simulink model "NCarState"  (R2024b)
settings: Solver=FixedStepDiscrete  StartTime=0.0  StopTime=1  FixedStep=0.001  RelTol=1e-3  EnableMultiTasking=on
settings Model: DataDictionary=Master_Dictionary.sldd  EnableAccessToBaseWorkspace=off  Creator=torni  LastModifiedBy=oxbro
settings SolverCC: AlgebraicLoopSolver=TrustRegion
settings DataIOCC: ReturnWorkspaceOutputs=off
settings OptimizationCC: DefaultParameterBehavior=Inlined  EnhancedBackFolding=on  PassReuseOutputArgsAs=Individual arguments  ZeroExternalMemoryAtStartup=off  ZeroInternalMemoryAtStartup=off  MaxStackSize=512  OptimizeBlockOrder=speed  DifferentSizesBufferReuse=on  OptimizationCustomize=off  EfficientTunableParamExpr=on
settings DebuggingCC: ParameterTunabilityLossMsg=error  UnconnectedInputMsg=warning  UnconnectedOutputMsg=warning  UnconnectedLineMsg=warning  ArithmeticOperatorsInVariantConditions=warning
settings HardwareCC: ProdBitPerPointer=32  ProdBitPerSizeT=32  ProdBitPerPtrDiffT=32  ProdLargestAtomicInteger=Long  ProdLargestAtomicFloat=Double  ProdWordSize=32  ProdLongLongMode=on  ProdHWDeviceType=ARM Compatible->ARM Cortex-M
settings ModelReferenceCC: EnableRefExpFcnMdlSchedulingChecks=on
settings SFSimCC: MATLABDynamicMemAlloc=off  CustomCodeUndefinedFunction=UseInterfaceOnly
settings RTWCC: Description=Embedded Coder  SystemTargetFile=ert.tlc  HardwareBoard=STM32H7xx Based (Single-core)  TemplateMakefile=ert_default_tmf  CustomHeaderCode="#include \"stm32h7xx_ll_tim.h\""  CustomInitializer=LL_TIM_EnableCounter(TIM2);  Toolchain=GNU Tools for ARM Embedded Processors  GPUComputeCapability=3.5
settings CodeAppCC: ForceParamTrailComments=on  IgnoreCustomStorageClasses=off  OperatorAnnotations=on  SimulinkDataObjDesc=on  SFDataObjDesc=on  InsertBlockDesc=on
settings ERTTargetCC: TargetLangStandard=C99 (ISO)  CodeReplacementLibrary=ARM Cortex-M  ExtModeTransport=3  ExtModeStaticAlloc=on  ExtModeStaticAllocSize=2048  ExtModeMexFile=ext_xcp  ExtModeIntrfLevel=Level2 - Open

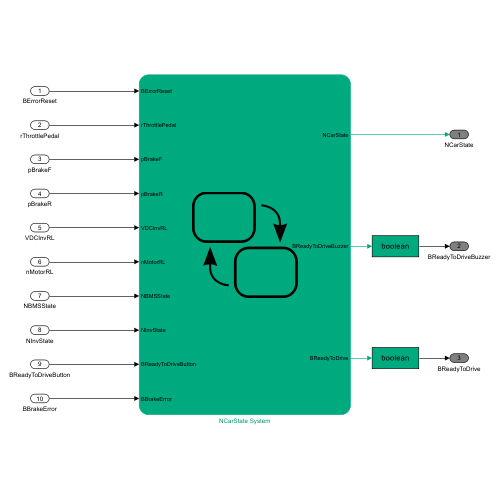
[thumbnail: Simulink's stored preview of the top-level diagram]
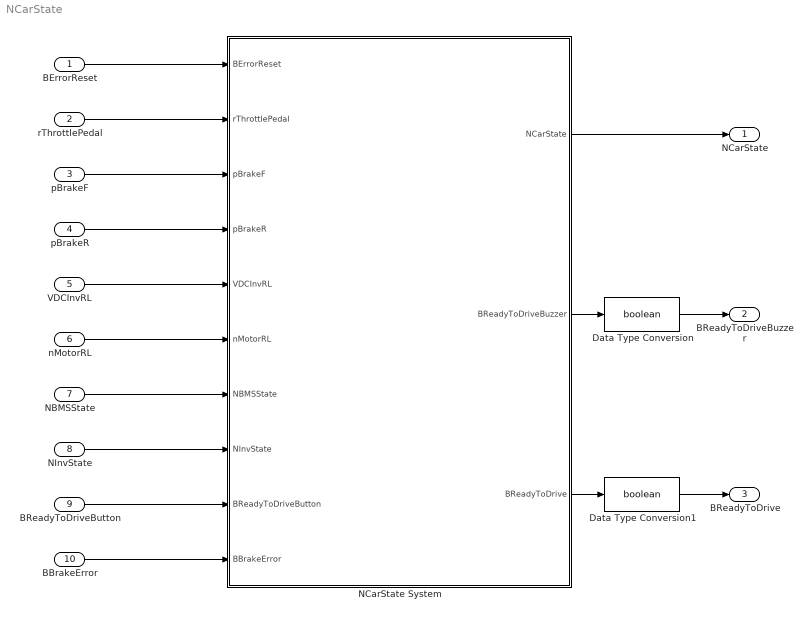
== system NCarState ==
  "BErrorReset " : Inport  OutDataTypeStr=boolean
  "rThrottlePedal " : Inport  Port=2  OutDataTypeStr=double
  "pBrakeF " : Inport  Port=3  OutDataTypeStr=double
  "pBrakeR " : Inport  Port=4  OutDataTypeStr=double
  VDCInvRL : Inport  Port=5  OutDataTypeStr=double
  "nMotorRL " : Inport  Port=6  OutDataTypeStr=double
  NBMSState : Inport  Port=7  OutDataTypeStr=double
  NInvState : Inport  Port=8  OutDataTypeStr=double
  BReadyToDriveButton : Inport  Port=9  OutDataTypeStr=boolean
  BBrakeError : Inport  Port=10  OutDataTypeStr=boolean
  Data Type Conversion : DataTypeConversion  OutDataTypeStr=boolean  SaturateOnIntegerOverflow=off  RndMeth=Floor
  Data Type Conversion1 : DataTypeConversion  OutDataTypeStr=boolean  SaturateOnIntegerOverflow=off  RndMeth=Floor
  NCarState System : Stateflow chart  TreatAsAtomicUnit=on
  NCarState : Outport  OutDataTypeStr=double  VectorParamsAs1DForOutWhenUnconnected=off
  BReadyToDriveBuzzer : Outport  Port=2  OutDataTypeStr=boolean  VectorParamsAs1DForOutWhenUnconnected=off
  BReadyToDrive : Outport  Port=3  OutDataTypeStr=boolean  VectorParamsAs1DForOutWhenUnconnected=off
  wires:
  "nMotorRL "/1 -> NCarState System/6(nMotorRL)
  "BErrorReset "/1 -> NCarState System/1(BErrorReset)
  "rThrottlePedal "/1 -> NCarState System/2(rThrottlePedal)
  "pBrakeR "/1 -> NCarState System/4(pBrakeR)
  VDCInvRL/1 -> NCarState System/5(VDCInvRL)
  "pBrakeF "/1 -> NCarState System/3(pBrakeF)
  NBMSState/1 -> NCarState System/7(NBMSState)
  NInvState/1 -> NCarState System/8(NInvState)
  NCarState System/2(BReadyToDriveBuzzer) -> Data Type Conversion/1
  NCarState System/3(BReadyToDrive) -> Data Type Conversion1/1
  Data Type Conversion/1 -> BReadyToDriveBuzzer/1
  Data Type Conversion1/1 -> BReadyToDrive/1
  BReadyToDriveButton/1 -> NCarState System/9(BReadyToDriveButton)
  NCarState System/1(NCarState) -> NCarState/1
  BBrakeError/1 -> NCarState System/10(BBrakeError)

== stateflow chart NCarState/NCarState System ==
  state Car_ON
    entry:
    NCarState=92;
    state ON
      entry:
      BReadyToDrive=1;
    (default) -> ON
  state Car_Idle_1
    entry:
    NCarState=0
    BReadyToDrive=0;
  state Status_Check1
    entry:
    NCarState=1;
  state BMS_Status_OK
    entry:
    NCarState=2
    BReadyToDrive=0;
  state Ready_To_Drive
    state RTD1
      entry:
      NCarState=6
      BReadyToDriveBuzzer=0
    state RTD_Sound
      entry:
      NCarState=5
      BReadyToDriveBuzzer=1
    RTD_Sound -> RTD1 : after(1500,tick)
    (default) -> RTD_Sound
  state Inv_LV_OK
    entry:
    NCarState=3
    BReadyToDrive=0;
  state Inv_HV_OK
    entry:
    NCarState=4;
  (default) -> Car_Idle_1
  Car_Idle_1 -> Status_Check1 : after(7000, tick)
  Status_Check1 -> BMS_Status_OK : after(500,tick)
      | [NBMSState == 92]
  Car_ON -> BMS_Status_OK : [VDCInvRL<60]
  RTD1 -> Car_ON : [rThrottlePedal<=5]
  Inv_HV_OK -> BMS_Status_OK [order 1] : [(BErrorReset==1 &&...
      | nMotorRL<500) ||...
      | (VDCInvRL<60)]
  Ready_To_Drive -> BMS_Status_OK : [VDCInvRL<60]
  BMS_Status_OK -> Inv_LV_OK : [NInvState == 3]
  Inv_LV_OK -> Inv_HV_OK : [NInvState == 92]
  Inv_HV_OK -> Ready_To_Drive [order 2] : [NInvState == 92 &&...
      | rThrottlePedal<=5 &&...
      | BReadyToDriveButton==1 &&...
      | pBrakeF >= 3 &&...
      | pBrakeR >= 3 &&...
      | BBrakeError <= 0.5]
  data: BErrorReset input boolean; NCarState output double; rThrottlePedal input double; pBrakeF input double; pBrakeR input double; VDCInvRL input double; nMotorRL input double; BReadyToDriveBuzzer output double; BReadyToDrive output double =0; NBMSState input double; NInvState input double; BReadyToDriveButton input boolean; BBrakeError input boolean
